simulink model "PredicteurDeSmith"  (R2015a)
settings: Solver=ode45  StartTime=0.0  StopTime=20.0  RelTol=1e-8
values from neighbouring files (symbols this model uses):
  ex1 = expm(m.ee(2).a*h)    [SpectreFini_script.m]
  h = lsim(m.ee,u,t)    [Modeles.m]    (also in Parametres.m = 0.06)
  K = place(m.ee(2).a,m.ee(2).b,vp_desirees)    [SpectreFini_script.m]
  km = 10    [Parametres.m]
  kr = 1/9    (= 0.111111111111)    [Parametres.m]
  ks = 10    [Parametres.m]
  taum = 0.3    [Parametres.m]
undefined symbols (not defined in the file or in its folder): m
libraries: dspmtrx3 x2
settings Model: Creator=Lucien  LastModifiedBy=Lucien

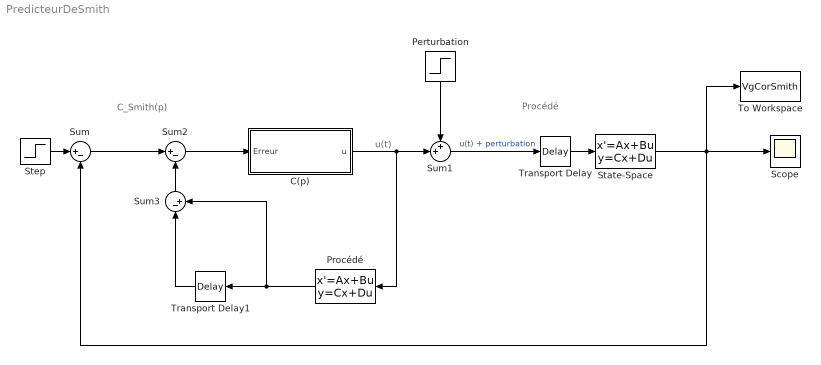
== system PredicteurDeSmith ==
  note: u(t)
  note: C_Smith(p)
  note: Procédé
  C(p) : Subsystem
  Perturbation : Step  Time=rand(1,1)*5  After=0  SampleTime=0
  Procédé : StateSpace  A=m.ee(2).a  B=m.ee(2).b  C=m.ee(2).c  D=m.ee(2).d  X0=0
  Scope : Scope
  State-Space : StateSpace  A=m.ee(2).a  B=m.ee(2).b  C=m.ee(2).c  D=m.ee(2).d  X0=0
  Step : Step  Time=0  SampleTime=0
  Sum : Sum  Inputs=|+-
  Sum1 : Sum  Inputs=++|
  Sum2 : Sum  Inputs=|+-
  Sum3 : Sum  Inputs=|-+
  To Workspace : ToWorkspace  VariableName=VgCorSmith  SaveFormat=Structure With Time  SampleTime=-1
  Transport Delay : TransportDelay  DelayTime=h
  Transport Delay1 : TransportDelay  DelayTime=h
  wires:
  Sum1/1 -> Transport Delay/1  "u(t) + perturbation"
  Sum/1 -> Sum2/1
  Step/1 -> Sum/1
  State-Space/1 -> To Workspace/1, Sum/2, Scope/1
  Transport Delay/1 -> State-Space/1
  Perturbation/1 -> Sum1/1
  C(p)/1("u ") -> Sum1/2, Procédé/1
  Sum2/1 -> C(p)/1("Erreur ")
  Procédé/1 -> Transport Delay1/1, Sum3/2
  Transport Delay1/1 -> Sum3/1
  Sum3/1 -> Sum2/2

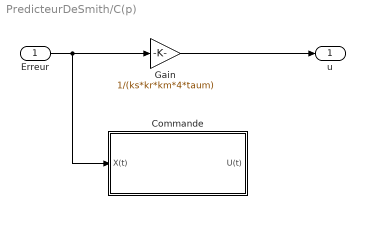
== system PredicteurDeSmith/C(p) ==
  "Erreur " : Inport
  Commande : Subsystem
  Gain : Gain  Gain=1/(ks*kr*km*4*taum)
  "u " : Outport
  wires:
  "Erreur "/1 -> Gain/1, Commande/1(X(t))
  Gain/1 -> "u "/1

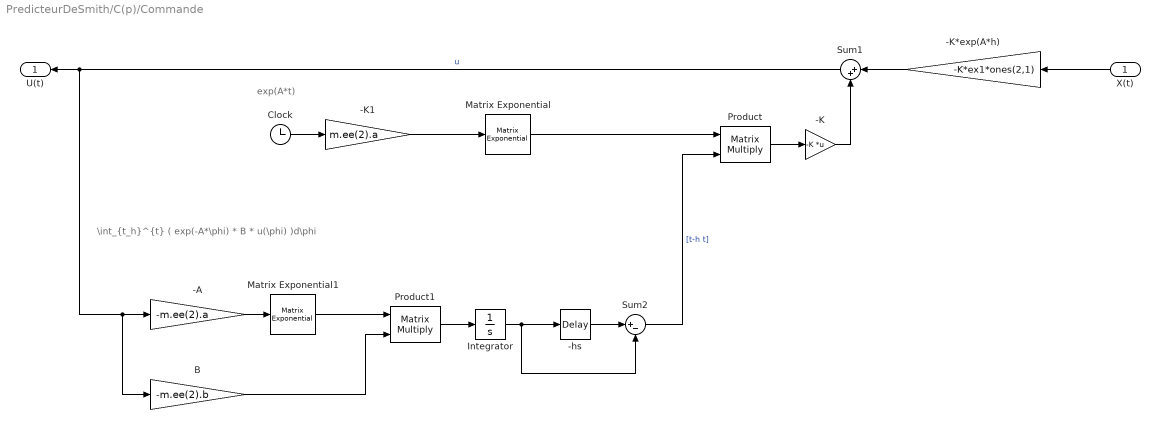
== system PredicteurDeSmith/C(p)/Commande ==
  note: \int_{t_h}^{t} ( exp(-A*\phi) * B * u(\phi) )d\phi
  note: exp(A*t)
  X(t) : Inport
  -A : Gain  Gain=-m.ee(2).a
  -K : Gain  Gain=-K  Multiplication=Matrix(K*u)
  -K*exp(A*h) : Gain  Gain=-K*ex1*ones(2,1)
  -K1 : Gain  Gain=m.ee(2).a
  -hs : TransportDelay  DelayTime=h
  B : Gain  Gain=-m.ee(2).b
  Clock : Clock
  Integrator : Integrator  AbsoluteTolerance=1e-6
  Matrix Exponential : dspmtrx3/Matrix Exponential
  Matrix Exponential1 : dspmtrx3/Matrix Exponential
  Product : Product  Multiplication=Matrix(*)
  Product1 : Product  Multiplication=Matrix(*)
  Sum1 : Sum  Inputs=|++
  Sum2 : Sum  Inputs=|+-
  U(t) : Outport
  wires:
  B/1 -> Product1/2
  Matrix Exponential1/1 -> Product1/1
  -K/1 -> Sum1/2
  X(t)/1 -> -K*exp(A*h)/1
  Sum1/1 -> U(t)/1, B/1, -A/1  "u"
  -K*exp(A*h)/1 -> Sum1/1
  -hs/1 -> Sum2/1
  Sum2/1 -> Product/2  "[t-h t]"
  Product1/1 -> Integrator/1
  Integrator/1 -> Sum2/2, -hs/1
  Matrix Exponential/1 -> Product/1
  Product/1 -> -K/1
  Clock/1 -> -K1/1
  -A/1 -> Matrix Exponential1/1
  -K1/1 -> Matrix Exponential/1
